simulink model "lstm_sim"  (R2023a)
settings: Solver=VariableStepAuto  StartTime=0.0  StopTime=t(end)  RelTol=1e-3
undefined symbols (not defined in the file): b, c0, F, h0, Nn, R, Ts, W
libraries: neural x5
settings Model: Creator=gcampa  LastModifiedBy=gcampa
settings DataIOCC: SaveFormat=Array  SaveOutput=off  SignalLogging=off  DSMLogging=off  SaveTime=off  ReturnWorkspaceOutputs=off
settings OptimizationCC: ReuseModelBlockBuffer=off

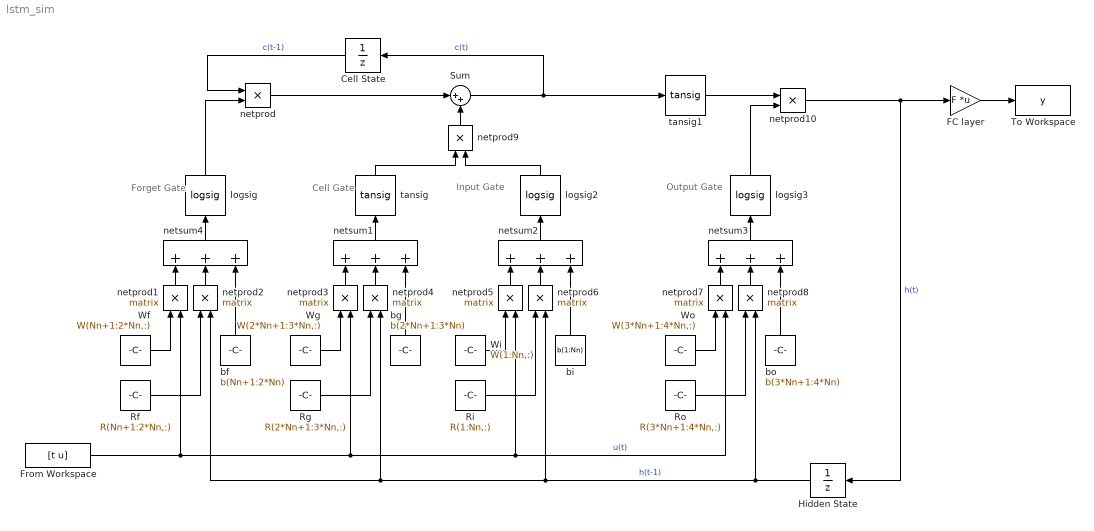
== system lstm_sim ==
  note: Forget
      | Gate
  note: Cell
      | Gate
  note: Input
      | Gate
  note: Output
      | Gate
  Cell State : UnitDelay  InitialCondition=c0  SampleTime=Ts  HasFrameUpgradeWarning=on
  FC layer : Gain  Gain=F  Multiplication=Matrix(K*u)
  From Workspace : FromWorkspace  VariableName=[t u]
  Hidden State : UnitDelay  InitialCondition=h0  SampleTime=Ts  HasFrameUpgradeWarning=on
  Rf : Constant  Value=R(Nn+1:2*Nn,:)
  Rg : Constant  Value=R(2*Nn+1:3*Nn,:)
  Ri : Constant  Value=R(1:Nn,:)
  Ro : Constant  Value=R(3*Nn+1:4*Nn,:)
  Sum : Sum  Inputs=|++
  To Workspace : ToWorkspace  VariableName=y  SampleTime=-1
  Wf : Constant  Value=W(Nn+1:2*Nn,:)
  Wg : Constant  Value=W(2*Nn+1:3*Nn,:)
  Wi : Constant  Value=W(1:Nn,:)
  Wo : Constant  Value=W(3*Nn+1:4*Nn,:)
  bf : Constant  Value=b(Nn+1:2*Nn)
  bg : Constant  Value=b(2*Nn+1:3*Nn)
  bi : Constant  Value=b(1:Nn)
  bo : Constant  Value=b(3*Nn+1:4*Nn)
  logsig : neural/Transfer Functions/logsig
  logsig2 : neural/Transfer Functions/logsig
  logsig3 : neural/Transfer Functions/logsig
  netprod : Product  InputSameDT=on  RndMeth=Zero  OutDataTypeStr=Inherit: Same as first input
  netprod{1..8} (8 alike) : Product  Multiplication=Matrix(*)  InputSameDT=on  RndMeth=Zero  SaturateOnIntegerOverflow=on  OutDataTypeStr=Inherit: Same as first input
  netprod10 : Product  InputSameDT=on  RndMeth=Zero  OutDataTypeStr=Inherit: Same as first input
  netprod9 : Product  InputSameDT=on  RndMeth=Zero  OutDataTypeStr=Inherit: Same as first input
  netsum{1..4} (4 alike) : Sum  Inputs=+++  InputSameDT=on  SaturateOnIntegerOverflow=on  OutDataTypeStr=Inherit: Same as first input
  tansig : neural/Transfer Functions/tansig
  tansig1 : neural/Transfer Functions/tansig
  wires:
  logsig/1 -> netprod/2
  netprod/1 -> Sum/1
  netsum4/1 -> logsig/1
  netsum1/1 -> tansig/1
  tansig/1 -> netprod9/1
  logsig2/1 -> netprod9/2
  netprod10/1 -> FC layer/1, Hidden State/1  "h(t)"
  Ro/1 -> netprod8/1
  netprod7/1 -> netsum3/1
  netsum3/1 -> logsig3/1
  Wo/1 -> netprod7/1
  logsig3/1 -> netprod10/2
  netprod9/1 -> Sum/2
  Sum/1 -> Cell State/1, tansig1/1  "c(t)"
  FC layer/1 -> To Workspace/1
  Cell State/1 -> netprod/1  "c(t-1)"
  netprod8/1 -> netsum3/2
  bo/1 -> netsum3/3
  bi/1 -> netsum2/3
  netprod6/1 -> netsum2/2
  Wi/1 -> netprod5/1
  netsum2/1 -> logsig2/1
  netprod5/1 -> netsum2/1
  Ri/1 -> netprod6/1
  Rg/1 -> netprod4/1
  netprod3/1 -> netsum1/1
  Wg/1 -> netprod3/1
  netprod4/1 -> netsum1/2
  bg/1 -> netsum1/3
  From Workspace/1 -> netprod1/2, netprod3/2, netprod7/2, netprod5/2  "u(t)"
  bf/1 -> netsum4/3
  netprod2/1 -> netsum4/2
  Hidden State/1 -> netprod2/2, netprod4/2, netprod6/2, netprod8/2  "h(t-1)"
  Wf/1 -> netprod1/1
  netprod1/1 -> netsum4/1
  Rf/1 -> netprod2/1
  tansig1/1 -> netprod10/1
